simulink model "softmodel"  (R2017a)
settings: Solver=ode8  StartTime=0.0  StopTime=25  FixedStep=0.001  MaxStep=0.01  RelTol=1e-3  AbsTol=1E-6  EnableMultiTasking=on
libraries: simulink x2
Description:
  | Bouncing Ball Model
  | 
  | This model calculates the trajectory, over time, of a ball thrown
  | upward with a velocity of 15 meters per second from a height of 10 m.
  | The model demonstrates the use of the 'ReinitDXDTwhenXreachesSaturation'
  | parameter in the Second-Order Integrator block to model this system.
  | This parameter, when set to 'on', forces a reinitialization of dx/dt
  | (velocity in the model) at the instant when x (position) reaches
  | saturation (i.e., when the ball hits the ground). The reinitialized value
  | is calculated by multiplying a coefficient of restitution times the ball
  | velocity, the instant before the ball hits the ground. The Memory block
  | in the calculation loop serves to capture the velocity of the ball just
  | before it hits the ground. The position of the ball is plotted in the
  | upper axis of the scope while the velocity of the ball is plotted in
  | the lower axis.
settings Model: Creator=The MathWorks, Inc.  LastModifiedBy=wangc
settings DataIOCC: MaxDataPoints=7500  SaveFormat=Array  SaveOutput=off  SignalLogging=off  DSMLogging=off  SaveTime=off
settings OptimizationCC: ExpressionDepthLimit=2147483647  EfficientFloat2IntCast=on  LifeSpan=inf
settings DebuggingCC: UnderspecifiedInitializationDetection=Classic  MergeDetectMultiDrivingBlocksExec=none  IgnoredZcDiagnostic=none  ParameterPrecisionLossMsg=none  FcnCallInpInsideContextMsg=warning  StateNameClashWarn=warning  SFUnexpectedBacktrackingDiag=warning  SFNoUnconditionalDefaultTransitionDiag=warning  SFExecutionAtInitializationDiag=none
settings HardwareCC: ProdBitPerPointer=32  ProdBitPerSizeT=32  ProdBitPerPtrDiffT=32  ProdLargestAtomicFloat=None  ProdIntDivRoundTo=Undefined  ProdEndianess=Unspecified  ProdWordSize=32  ProdHWDeviceType=32-bit Generic  TargetBitPerPointer=64  TargetBitPerSizeT=64  TargetBitPerPtrDiffT=64  TargetLongLongMode=on  TargetIntDivRoundTo=Zero  TargetEndianess=LittleEndian  TargetWordSize=64  TargetHWDeviceType=MATLAB Host  ProdEqTarget=off
settings ModelReferenceCC: PropagateSignalLabelsOutOfModel=off
settings RTWCC: SystemTargetFile=rsim.tlc  TemplateMakefile=rsim_default_tmf  Description=Rapid Simulation Target
settings ConfigComp: CovMetricSettings=dw  CovHtmlReporting=on  CovSaveCumulativeToWorkspaceVar=on  CovSaveSingleToWorkspaceVar=on  CovExternalEMLEnable=off

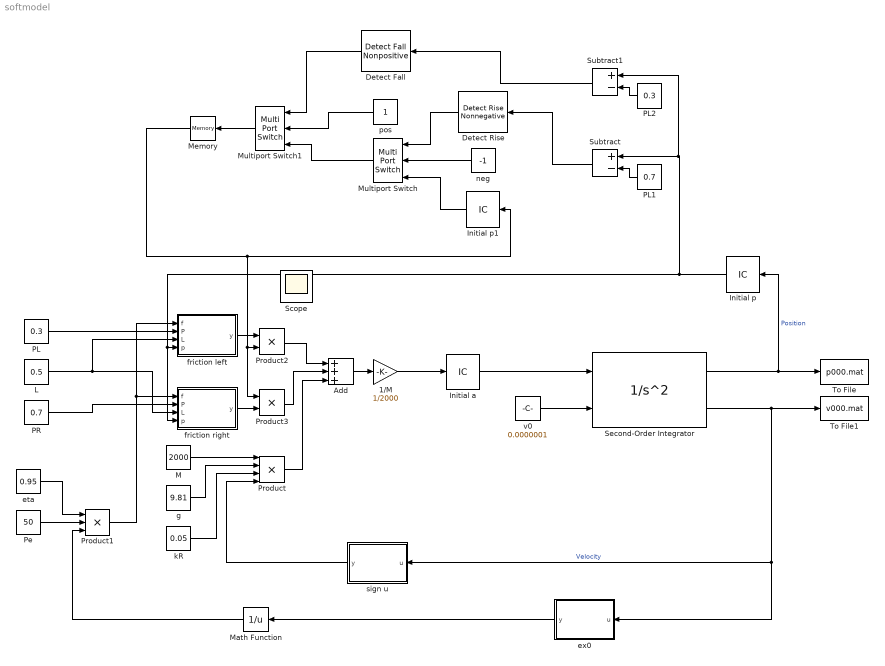
== system softmodel ==
  1/M : Gain  Gain=1/2000
  Add : Sum  Inputs=3
  Detect Fall : simulink/Logic and Bit Operations/Detect Fall Nonpositive  vinit=0.25  OutDataTypeStr=boolean
      settings: SourceProductName=Simulink  SourceProductBaseCode=SL
  Detect Rise : simulink/Logic and Bit Operations/Detect Rise Nonnegative  vinit=0.25  OutDataTypeStr=boolean
      settings: SourceProductName=Simulink  SourceProductBaseCode=SL
  Initial a : InitialCondition  Value=0
  Initial p : InitialCondition  Value=0.3
  Initial p1 : InitialCondition
  L : Constant  Value=0.5
  M : Constant  Value=2000
  Math Function : Math  Operator=reciprocal  SaturateOnIntegerOverflow=on
  Memory : Memory  X0=1
  Multiport Switch : MultiPortSwitch  DataPortOrder=Specify indices  Inputs=2  DataPortIndices={1,0}
  Multiport Switch1 : MultiPortSwitch  DataPortOrder=Specify indices  Inputs=2  DataPortIndices={1,0}
  PL : Constant  Value=0.3
  PL1 : Constant  Value=0.7
  PL2 : Constant  Value=0.3
  PR : Constant  Value=0.7
  Pe : Constant  Value=50
  Product : Product  Inputs=4
  Product1 : Product  Inputs=3
  Product2 : Product
  Product3 : Product
  Second-Order Integrator : SecondOrderIntegrator  ICX=0.25  LimitX=on  UpperLimitX=1  LowerLimitX=0  StateNameX='Position'  ICSourceDXDT=external  StateNameDXDT='Velocity'  ZeroCross=off
  Subtract : Sum  Inputs=+-
  Subtract1 : Sum  Inputs=+-
  To File : ToFile  Filename=p000.mat  MatrixName=p  SaveFormat=Timeseries
  To File1 : ToFile  Filename=v000.mat  MatrixName=v  SaveFormat=Timeseries
  eta : Constant  Value=0.95
  ex0 : MATLAB Function  TreatAsAtomicUnit=on
  friction left : MATLAB Function  TreatAsAtomicUnit=on
  friction right : MATLAB Function  TreatAsAtomicUnit=on
  g : Constant  Value=9.81
  kR : Constant  Value=0.05
  neg : Constant  Value=-1
  pos : Constant
  sign u : MATLAB Function  TreatAsAtomicUnit=on
  v0 : Constant  Value=0.0000001
  Scope : Scope
  wires:
  Initial a/1 -> Second-Order Integrator/1
  Second-Order Integrator/1 -> To File/1, Initial p/1  "Position"
  Second-Order Integrator/2 -> To File1/1, sign u/1(u), ex0/1(u)  "Velocity"
  v0/1 -> Second-Order Integrator/2
  M/1 -> Product/1
  g/1 -> Product/2
  kR/1 -> Product/3
  friction left/1(y) -> Product2/1
  friction right/1(y) -> Product3/2
  Product/1 -> Add/3
  Add/1 -> 1/M/1
  1/M/1 -> Initial a/1
  Initial p/1 -> friction right/4(p), friction left/4(p), Subtract1/1, Subtract/1
  eta/1 -> Product1/1
  Pe/1 -> Product1/2
  Product1/1 -> friction right/1(f), friction left/1(f)
  PL/1 -> friction left/2(P)
  L/1 -> friction right/3(L), friction left/3(L)
  PR/1 -> friction right/2(P)
  sign u/1(y) -> Product/4
  Product2/1 -> Add/1
  Product3/1 -> Add/2
  Memory/1 -> Product3/1, Product2/2, Initial p1/1
  PL1/1 -> Subtract/2
  Detect Rise/1 -> Multiport Switch/1
  neg/1 -> Multiport Switch/2
  Initial p1/1 -> Multiport Switch/3
  Multiport Switch/1 -> Multiport Switch1/3
  pos/1 -> Multiport Switch1/2
  Detect Fall/1 -> Multiport Switch1/1
  Multiport Switch1/1 -> Memory/1
  Subtract/1 -> Detect Rise/1
  PL2/1 -> Subtract1/2
  Subtract1/1 -> Detect Fall/1
  ex0/1(y) -> Math Function/1
  Math Function/1 -> Product1/3

== matlab function softmodel/friction right ==
  data: f input; P input; L input; y output; p input
function y = fcn(f,P,L,p)
    % f 驱动力
    % p 滑板位置
    % P 驱动位置
    y = f.*(p>=P-L/2 & p<=P+L/2)+0;

== matlab function softmodel/friction left ==
  data: f input; P input; L input; y output; p input
function y = fcn(f,P,L,p)
    % f 驱动力
    % p 滑板位置
    % P 驱动位置
    y = f.*(p>=P-L/2 & p<=P+L/2)+0;

== matlab function softmodel/sign u ==
  data: u input; y output
function y = fcn(u)

y = -1*sign(u);

== matlab function softmodel/ex0 ==
  data: u input; y output
function y = fcn(u)
upper=0.001
lower=-1*upper

y = abs(u).*(u>=upper|u<=lower)+upper.*(u<upper & u>lower);
